simulink model "RotatingMasses_Template"  (R2019b)
settings: Solver=ode1  StartTime=0.0  StopTime=110  FixedStep=0.002  RelTol=1e-3  EnableMultiTasking=on
PostLoadFcn:
  | qc_set_target_type(getConfigSet(bdroot, 'QUARC Default Target Configuration'));
values from neighbouring files (symbols this model uses):
  data = dataset_struct    [create_data.m]    (also in data_loader.m = [])
  deg_to_rad = pi/180    (= 0.0174532925199)    [sensors_parameters.m]
  experiment = merge( experiment, experiment2 )    [blackbox_est.m]    (also in experiment_handler.m = obj.experiments{idx_exp}; guided_script.m = e_h.experiments{40}; test_controllori.m = e_h.load_experiment)
  pulse_to_rad = 2*pi/pulse_per_rev_encoder    (= 0.00153398078789)    [sensors_parameters.m]
  V_th = V_max*1    [sensors_parameters.m]
  Vmin_pot = -4.8924    [sensors_parameters.m]
  volt_to_deg_potentiometer = 352/(Vmax_pot-Vmin_pot)    (= 36.7512711555)    [sensors_parameters.m]
undefined symbols (not defined in the file or in its folder): controller, HIL, qc_get_step_size
libraries: simulink x43, cstblocks x15, quarc_library x5
(part 1 of 3)
settings Model: SimulationMode=external  ExtModeTrigDuration=5000  Creator=CFulford  LastModifiedBy=denniszanutto
settings SolverCC: PositivePriorityOrder=on
settings DataIOCC: LimitDataPoints=on  SaveFormat=Array  SignalLoggingSaveFormat=ModelDataLogs  ReturnWorkspaceOutputs=off
settings OptimizationCC: ExpressionDepthLimit=2147483647  InitFltsAndDblsToZero=on  LifeSpan=inf
settings DebuggingCC: SaveWithParameterizedLinksMsg=none  UnderspecifiedInitializationDetection=Classic  MergeDetectMultiDrivingBlocksExec=none  SolverPrmCheckMsg=warning  MultiTaskDSMMsg=warning  MultiTaskCondExecSysMsg=none  FcnCallInpInsideContextMsg=warning  StateNameClashWarn=warning  SFUnexpectedBacktrackingDiag=warning  SFNoUnconditionalDefaultTransitionDiag=warning  SFExecutionAtInitializationDiag=none  ArithmeticOperatorsInVariantConditions=warning
settings HardwareCC: ProdBitPerPointer=32  ProdBitPerSizeT=32  ProdBitPerPtrDiffT=32  ProdLargestAtomicFloat=None  ProdIntDivRoundTo=Undefined  ProdEndianess=Unspecified  ProdWordSize=32  ProdHWDeviceType=32-bit Generic
settings ModelReferenceCC: PropagateSignalLabelsOutOfModel=off
settings SFSimCC: SimUseLocalCustomCode=off  CustomCodeUndefinedFunction=UseInterfaceOnly
settings RTWCC: Description=QUARC Win64 Target  SystemTargetFile=quarc_win64.tlc  TemplateMakefile=quarc_default_tmf  RTWUseLocalCustomCode=off
settings CodeAppCC: StateflowObjectComments=on
settings STFCustomTargetCC: TargetPreCompLibLocation=C:\PROGRA~3\QUARC\lib\2019b\win64\release  ConcurrentExecutionCompliant=on  GeneratePreprocessorConditionals=Disable all  CombineOutputUpdateFcns=on  CPPClassGenCompliant=on  SystemTargetFile=quarc_win64.tlc
settings GRTTargetCC: TargetPreCompLibLocation=C:\PROGRA~3\QUARC\lib\2019b\win64\release  TargetLangStandard=C89/C90 (ANSI)  ParMdlRefBuildCompliant=off  CompOptLevelCompliant=off  GeneratePreprocessorConditionals=Disable all  MatFileLogging=off  UseToolchainInfoCompliant=off  ExtMode=on  ExtModeMexFile=quarc_comm
settings ConfigComp: CovMetricSettings=dw  CovHtmlReporting=on  CovSaveCumulativeToWorkspaceVar=on  CovSaveSingleToWorkspaceVar=on  CovExternalEMLEnable=off  CovSFcnEnable=off

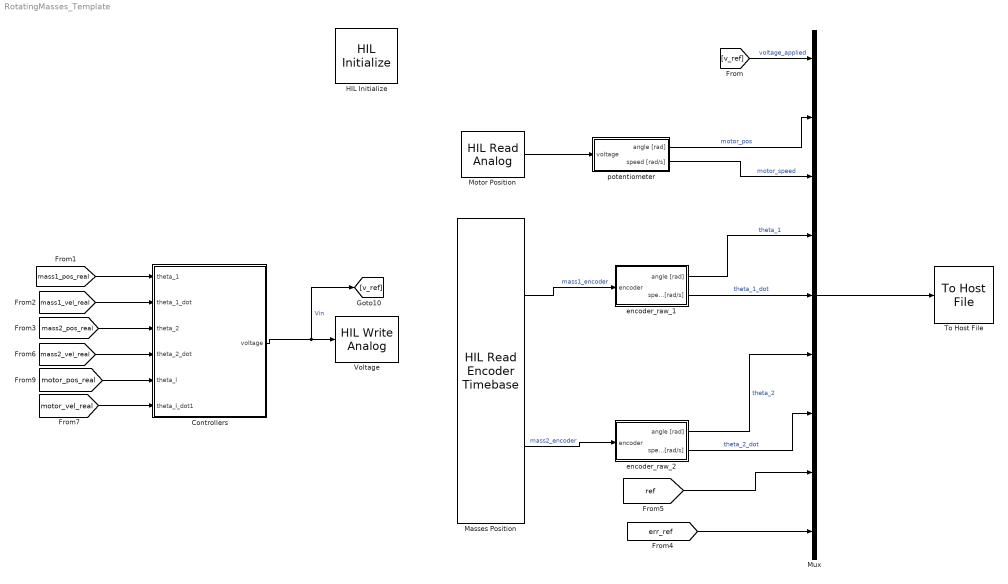
== system RotatingMasses_Template ==
  Controllers : Subsystem
  HIL Initialize : quarc_library/Data Acquisition/Generic/Configuration/HIL Initialize  Priority=-99  object_name=HIL-1  board_type=q2_usb  board_number=0  board_options=d0=digital;d1=digital;led=auto;update_rate=normal;decimation=1  exclusive=off  active=off  hardware_clocks=[0]  clock_modes=[]  initial_clock_frequencies=[]  set_clock_params_at_start=off  set_clock_params_at_switch_in=off  set_clock_frequencies_at_start=off  set_clock_frequencies_at_switch_in=off  analog_input_channels=[0:1]  analog_input_configurations=[]  analog_input_maximums=10  analog_input_minimums=-10  set_analog_input_params_at_start=on  set_analog_input_params_at_switch_in=off  analog_output_channels=[0:1]  analog_output_maximums=10  analog_output_minimums=-10  initial_analog_outputs=[0]  final_analog_outputs=[0]  watchdog_analog_outputs=0  set_analog_output_params_at_start=on  set_analog_output_params_at_switch_in=off  set_analog_outputs_at_start=on  set_analog_outputs_at_switch_in=off  set_analog_outputs_at_terminate=on  set_analog_outputs_at_switch_out=off  set_analog_outputs_on_watchdog=off  digital_input_channels=[]  digital_output_channels=[]  digital_output_configuration=[]  initial_digital_outputs=[1]  final_digital_outputs=[1]  watchdog_digital_outputs=[1]  set_digital_output_params_at_start=off  set_digital_output_params_at_switch_in=off  set_digital_outputs_at_start=on  set_digital_outputs_at_switch_in=off  set_digital_outputs_at_terminate=on  set_digital_outputs_at_switch_out=off  set_digital_outputs_on_watchdog=off  encoder_channels=[0:1]  quadrature=[4]  encoder_filter_frequency=[]  initial_encoder_counts=[0]  set_encoder_params_at_start=on  set_encoder_params_at_switch_in=off  set_encoder_counts_at_start=on  set_encoder_counts_at_switch_in=off  pwm_channels=[]  pwm_modes=[0]  pwm_frequency=1/0.020  pwm_configuration=[]  pwm_alignment=[]  pwm_polarity=[]  pwm_leading_deadband=[]  pwm_trailing_deadband=[]  initial_pwm_outputs=[0]  final_pwm_outputs=[0]  watchdog_pwm_outputs=[0]  set_pwm_params_at_start=on  set_pwm_params_at_switch_in=off  set_pwm_outputs_at_start=on  set_pwm_outputs_at_switch_in=off  set_pwm_outputs_at_terminate=on  set_pwm_outputs_at_switch_out=off  set_pwm_outputs_on_watchdog=off  other_output_channels=[]  initial_other_outputs=[]  final_other_outputs=[]  watchdog_other_outputs=[]  set_other_outputs_at_start=off  set_other_outputs_at_switch_in=off  set_other_outputs_at_terminate=off  set_other_outputs_at_switch_out=off  set_other_outputs_on_watchdog=off
  Masses Position : quarc_library/Data Acquisition/Generic/Timebases/HIL Read Encoder Timebase  object_name=HIL-1  clock=0  channels=[0:1]  samples_in_buffer=max(ceil(1/qc_get_step_size), 1)  active=on  vector_output=off  data_type_mode=Inherit via back propagation  data_type=double
  Motor Position : quarc_library/Data Acquisition/Generic/Immediate I//O/HIL Read Analog  object_name=HIL-1  channels=0  sample_time=qc_get_step_size  active=on  vector_output=off
  Mux : Mux  Inputs=9
  To Host File : quarc_library/Sinks/To Host/To Host File  file_name=data_%{date}_%{time}.mat  variable_name=data_%{date}_%{time}  decimation=1  sample_time=-1  file_format=MAT-file v.5  options=No header or footer  append=off  final_file_name=data_04-May-2021_18-47-16.mat  bitrate=2000000
  Voltage : quarc_library/Data Acquisition/Generic/Immediate I//O/HIL Write Analog  object_name=HIL-1  channels=0  sample_time=-1  active=off  vector_input=off
  encoder_raw_1 : Subsystem
  encoder_raw_2 : Subsystem
  potentiometer : Subsystem
  wires:
  potentiometer/1(angle [rad]) -> Mux/2  "motor_pos"
  Mux/1 -> To Host File/1
  Motor Position/1 -> potentiometer/1(voltage)
  [v_ref] -> Mux/1  "voltage_applied"
  Masses Position/1 -> encoder_raw_1/1(encoder)  "mass1_encoder"
  encoder_raw_1/1("angle [rad] ") -> Mux/4  "theta_1"
  Masses Position/2 -> encoder_raw_2/1(encoder)  "mass2_encoder"
  [err_ref] -> Mux/9
  [ref] -> Mux/8
  ? -> ?
  encoder_raw_1/2(speed [rad/s]) -> Mux/5  "theta_1_dot"
  encoder_raw_2/1("angle [rad] ") -> Mux/6  "theta_2"
  encoder_raw_2/2(speed [rad/s]) -> Mux/7  "theta_2_dot"
  Controllers/1(voltage) -> Voltage/1, [v_ref]  "Vin"
  [mass1_pos_real] -> Controllers/1(theta_1)
  [mass1_vel_real] -> Controllers/2(theta_1_dot)
  [mass2_pos_real] -> Controllers/3(theta_2)
  [mass2_vel_real] -> Controllers/4(theta_2_dot)
  potentiometer/2(speed [rad/s]) -> Mux/3  "motor_speed"
  [motor_pos_real] -> Controllers/5(theta_l)
  [motor_vel_real] -> Controllers/6(theta_l_dot1)

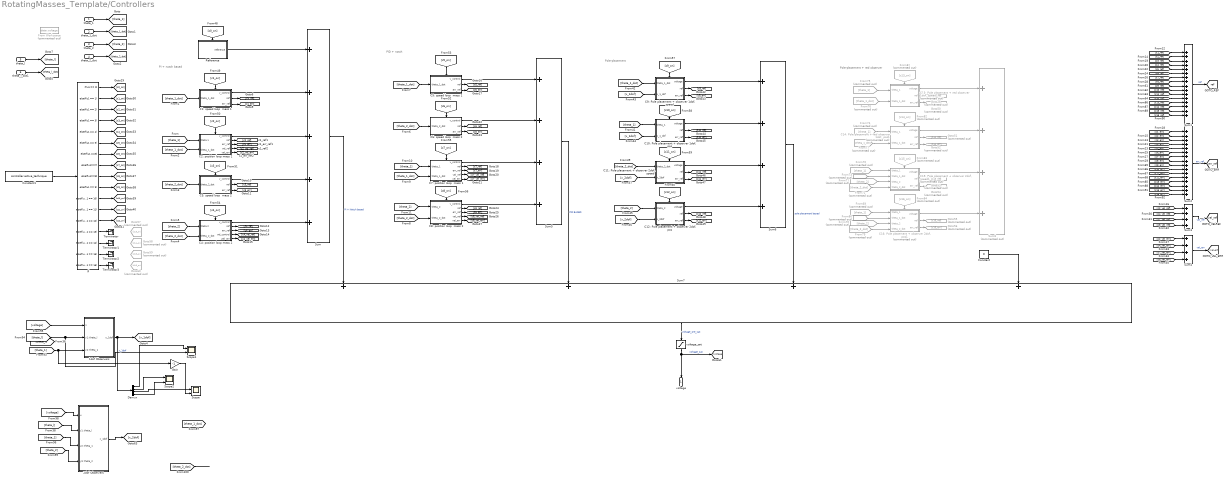
== system RotatingMasses_Template/Controllers ==
  note: Pole-placement
  note: PID + notch
  note: PI + notch based
  note: Pole-placement + red observer
  theta_1 : Inport
  theta_1_dot : Inport  Port=2
  theta_2 : Inport  Port=3
  theta_2_dot : Inport  Port=4
  theta_l : Inport  Port=5
  theta_l_dot1 : Inport  Port=6
  1dof Observers : Subsystem
  2dof Observers : Subsystem
  "C10: Pole placement + observer 1dof, pos" : Subsystem  TreatAsAtomicUnit=on
  "C11: Pole placement + observer 2dof, speed" : Subsystem  TreatAsAtomicUnit=on
  "C12: Pole placement + observer 2dof, pos" : Subsystem  TreatAsAtomicUnit=on
  "C13: Pole placement + red observer 1dof, speed1" : Subsystem  Commented=on  TreatAsAtomicUnit=on
  "C14: Pole placement + red observer 1dof, pos1" : Subsystem  Commented=on  TreatAsAtomicUnit=on
  "C15: Pole placement + observer 2dof, speed1" : Subsystem  Commented=on  TreatAsAtomicUnit=on
  "C16: Pole placement + observer 2dof, pos1" : Subsystem  Commented=on  TreatAsAtomicUnit=on
  C1: speed loop  mass 1 : Subsystem
  C2: position loop mass 1 : Subsystem
  C3: speed loop  mass 2 : Subsystem
  C4: position loop mass 2 : Subsystem
  C5: speed loop  mass 1 : Subsystem
  C6: speed loop  mass 2 : Subsystem
  C7: position loop  mass 1 : Subsystem
  C8: position loop  mass 2 : Subsystem
  "C9: Pole placement + observer 1dof, speed" : Subsystem  TreatAsAtomicUnit=on
  Constant : Constant  Value=0
  Constant1 : Constant  Value=controller.active_technique
  Demux : Demux
  From Workspace : FromWorkspace  Commented=on  VariableName=data.voltage  SampleTime=0
  From{69..70,74..75} (4 alike) : From  Commented=on  GotoTag=theta_1
  From71 : From  Commented=on  GotoTag=theta_2
  From72 : From  Commented=on  GotoTag=theta_2_dot
  From{73,76..77,80} (4 alike) : From  Commented=on  GotoTag=theta_1_dot
  From78 : From  Commented=on  GotoTag=theta_2
  From79 : From  Commented=on  GotoTag=theta_2_dot
  From81 : From  Commented=on  GotoTag=c13_on
  From82 : From  Commented=on  GotoTag=c14_on
  From83 : From  Commented=on  GotoTag=c15_on
  From84 : From  Commented=on  GotoTag=c16_on
  Gain : Gain  Gain=-1
  Goto28 : Goto  Commented=on  GotoTag=c13_ref
  Goto50 : Goto  Commented=on  GotoTag=c13_err
  Goto51 : Goto  Commented=on  GotoTag=c14_ref
  Goto52 : Goto  Commented=on  GotoTag=c14_err
  Goto53 : Goto  Commented=on  GotoTag=c15_ref
  Goto54 : Goto  Commented=on  GotoTag=c15_err
  Goto55 : Goto  Commented=on  GotoTag=c16_ref
  Goto56 : Goto  Commented=on  GotoTag=c16_err
  Goto57 : Goto  Commented=on  GotoTag=c13_on
  Goto58 : Goto  Commented=on  GotoTag=c14_on
  Goto59 : Goto  Commented=on  GotoTag=c15_on
  Goto60 : Goto  Commented=on  GotoTag=c16_on
  If : If  IfExpression=u1 == 0  ElseIfExpressions=u1 == 1, u1 == 2, u1 == 3, u1 == 4, u1 == 5, u1 ==6, u1==7, u1==8, u1 == 9, u1 == 10, u1 == 11, u1 == 12, u1 == 13, u1 == 14, u1 == 15, u1 == 16  ShowElse=off
  Reference : Subsystem
  Scope : Scope  NumInputPorts=2
  Scope1 : Scope  NumInputPorts=2
  Scope2 : Scope  NumInputPorts=2
  Sum : Sum  Inputs=+++++
  Sum1 : Sum  Inputs=++++++++++++++++
  Sum2 : Sum  Inputs=++++++++++++++++
  Sum{3..7} (5 alike) : Sum  Inputs=++++
  Sum8 : Sum  Commented=on  Inputs=++++
  Terminator{,1..3} (4 alike) : Terminator
  voltage_sat : Saturate  UpperLimit=V_th  LowerLimit=-V_th
  voltage : Outport
  tag scope: err_ref=global, ref=global, vel_ref=global
  wires:
  voltage_sat/1 -> voltage/1, [voltage]  "voltage_sat"
  theta_1_dot/1 -> [theta_1_dot]
  C4: position loop mass 2/1(v_control) -> Sum/5
  C3: speed loop  mass 2/1(v_control) -> Sum/4
  C2: position loop mass 1/1(v_control) -> Sum/3
  C1: speed loop  mass 1/1(v_control) -> Sum/2
  Reference/1(reference) -> Sum/1
  If/1 -> [c0_on]
  Constant1/1 -> If/1
  theta_1/1 -> [theta_1]
  [theta_1_dot] -> C1: speed loop  mass 1/1(theta_1_dot)
  [theta_1_dot] -> C2: position loop mass 1/2(theta_1_dot)
  [theta_1] -> C2: position loop mass 1/1(theta 1)
  theta_2_dot/1 -> [theta_2_dot]
  [theta_2_dot] -> C3: speed loop  mass 2/1(theta_2_dot)
  [theta_2_dot] -> C4: position loop mass 2/2(theta_2_dot)
  theta_2/1 -> [theta_2]
  [theta_2] -> C4: position loop mass 2/1(theta 2)
  [theta_2_dot] -> C6: speed loop  mass 2/1(theta_2_dot)
  C6: speed loop  mass 2/1(v_control) -> Sum5/2
  C5: speed loop  mass 1/1(v_control) -> Sum5/1
  [theta_1_dot] -> C5: speed loop  mass 1/1(theta_1_dot)
  C8: position loop  mass 2/1(v_control) -> Sum5/4
  [theta_1_dot] -> C7: position loop  mass 1/2(theta_1_dot)
  [theta_2_dot] -> C8: position loop  mass 2/2(theta_2_dot)
  C7: position loop  mass 1/1(v_control) -> Sum5/3
  [theta_1] -> C7: position loop  mass 1/1(theta_1)
  [theta_2] -> C8: position loop  mass 2/1(theta_2)
  C1: speed loop  mass 1/2("ref ") -> [c1_ref]
  C1: speed loop  mass 1/3("err_ref ") -> [c1_err]
  C2: position loop mass 1/5("vel_err ") -> [c2_vel_err]
  C2: position loop mass 1/4("vel_ref ") -> [c2_vel_ref]
  C2: position loop mass 1/3("err_ref ") -> [c2_err]
  C3: speed loop  mass 2/2("ref ") -> [c3_ref]
  C3: speed loop  mass 2/3("err_ref ") -> [c3_err]
  C4: position loop mass 2/3(err_ref) -> [c4_err]
  C4: position loop mass 2/2(ref) -> [c4_ref]
  C4: position loop mass 2/4(vel_control) -> [c4_vel_ref]
  C4: position loop mass 2/5("vell_err ") -> [c4_vel_err]
  C5: speed loop  mass 1/2("ref ") -> [c5_ref]
  C5: speed loop  mass 1/3("err_ref ") -> [c5_err]
  C7: position loop  mass 1/5(vel_err) -> [c7_vel_err]
  C7: position loop  mass 1/2("ref ") -> [c7_ref]
  C7: position loop  mass 1/3("err_ref ") -> [c7_err]
  C7: position loop  mass 1/4(vel_ref) -> [c7_vel_ref]
  C6: speed loop  mass 2/2("ref ") -> [c6_ref]
  C6: speed loop  mass 2/3("err_ref ") -> [c6_err]
  C8: position loop  mass 2/2("ref ") -> [c8_ref]
  C8: position loop  mass 2/3("err_ref ") -> [c8_err]
  C8: position loop  mass 2/4(vel_ref) -> [c8_vel_ref]
  C8: position loop  mass 2/5(vel_err) -> [c8_vel_err]
  [c1_ref] -> Sum1/1
  [c2_ref] -> Sum1/2
  Sum1/1 -> [ref]  "ref"
  [c1_err] -> Sum2/1
  Sum2/1 -> [err_ref]  "err_ref"
  [c2_err] -> Sum2/2
  C2: position loop mass 1/2("ref ") -> [c2_ref]
  [c3_err] -> Sum2/3
  [c3_ref] -> Sum1/3
  [c6_err] -> Sum2/6
  [c7_err] -> Sum2/7
  [c8_err] -> Sum2/8
  [c4_err] -> Sum2/4
  [c5_err] -> Sum2/5
  [c4_ref] -> Sum1/4
  [c5_ref] -> Sum1/5
  [c6_ref] -> Sum1/6
  [c8_ref] -> Sum1/8
  [c7_ref] -> Sum1/7
  [c8_vel_ref] -> Sum3/4
  [c7_vel_ref] -> Sum3/3
  [c4_vel_ref] -> Sum3/2
  [c2_vel_ref] -> Sum3/1
  Sum3/1 -> [vel_ref]  "vel_ref"
  [c2_vel_err] -> Sum4/1
  Sum4/1 -> [vel_err]  "vel_err"
  [c4_vel_err] -> Sum4/2
  [c7_vel_err] -> Sum4/3
  [c8_vel_err] -> Sum4/4
  [theta_2_dot] -> "C11: Pole placement + observer 2dof, speed"/1(theta_2_dot)
  "C9: Pole placement + observer 1dof, speed"/1(voltage) -> Sum6/1
  [theta_1_dot] -> "C9: Pole placement + observer 1dof, speed"/1(theta_1_dot)
  [x_1dof] -> "C9: Pole placement + observer 1dof, speed"/2(x_1_dof)
  [theta_1] -> "C10: Pole placement + observer 1dof, pos"/1(theta_1)
  [x_1dof] -> "C10: Pole placement + observer 1dof, pos"/2(x_1_dof)
  "C10: Pole placement + observer 1dof, pos"/1(voltage) -> Sum6/2
  "C11: Pole placement + observer 2dof, speed"/1(voltage) -> Sum6/3
  "C12: Pole placement + observer 2dof, pos"/1(voltage) -> Sum6/4
  [x_2dof] -> "C12: Pole placement + observer 2dof, pos"/2(x_2dof)
  [theta_2] -> "C12: Pole placement + observer 2dof, pos"/1(theta_2)
  [c0_on] -> Reference/Action
  If/2 -> [c1_on]
  [c1_on] -> C1: speed loop  mass 1/Action
  If/3 -> [c2_on]
  [c2_on] -> C2: position loop mass 1/Action
  If/4 -> [c3_on]
  [c3_on] -> C3: speed loop  mass 2/Action
  If/7 -> [c6_on]
  If/6 -> [c5_on]
  If/5 -> [c4_on]
  [c4_on] -> C4: position loop mass 2/Action
  [c5_on] -> C5: speed loop  mass 1/Action
  [c6_on] -> C6: speed loop  mass 2/Action
  If/8 -> [c7_on]
  [c7_on] -> C7: position loop  mass 1/Action
  If/9 -> [c8_on]
  [c8_on] -> C8: position loop  mass 2/Action
  If/10 -> [c9_on]
  [c9_on] -> "C9: Pole placement + observer 1dof, speed"/Action
  If/11 -> [c10_on]
  [c10_on] -> "C10: Pole placement + observer 1dof, pos"/Action
  If/12 -> [c11_on]
  [c11_on] -> "C11: Pole placement + observer 2dof, speed"/Action
  [c12_on] -> "C12: Pole placement + observer 2dof, pos"/Action
  If/13 -> [c12_on]
  "C9: Pole placement + observer 1dof, speed"/2(ref) -> [c9_ref]
  "C9: Pole placement + observer 1dof, speed"/3(err_ref) -> [c9_err]
  "C10: Pole placement + observer 1dof, pos"/2(ref) -> [c10_ref]
  "C10: Pole placement + observer 1dof, pos"/3(err_ref) -> [c10_err]
  "C11: Pole placement + observer 2dof, speed"/2(ref) -> [c11_ref]
  "C11: Pole placement + observer 2dof, speed"/3(err_ref) -> [c11_err]
  "C12: Pole placement + observer 2dof, pos"/2(ref) -> [c12_ref]
  "C12: Pole placement + observer 2dof, pos"/3(err_ref) -> [c12_err]
  [c9_ref] -> Sum1/9
  [c10_ref] -> Sum1/10
  [c11_ref] -> Sum1/11
  [c12_ref] -> Sum1/12
  [c9_err] -> Sum2/9
  [c10_err] -> Sum2/10
  [c11_err] -> Sum2/11
  [c12_err] -> Sum2/12
  "C15: Pole placement + observer 2dof, speed1"/3(err_ref) -> Goto54/1
  "C16: Pole placement + observer 2dof, pos1"/2(ref) -> Goto55/1
  From84/1 -> "C16: Pole placement + observer 2dof, pos1"/Action
  From71/1 -> "C15: Pole placement + observer 2dof, speed1"/3(theta_2)
  "C16: Pole placement + observer 2dof, pos1"/3(err_ref) -> Goto56/1
  "C13: Pole placement + red observer 1dof, speed1"/2(ref) -> Goto28/1
  From78/1 -> "C16: Pole placement + observer 2dof, pos1"/3(theta_2)
  From74/1 -> "C14: Pole placement + red observer 1dof, pos1"/1(theta_1)
  "C13: Pole placement + red observer 1dof, speed1"/3(err_ref) -> Goto50/1
  "C14: Pole placement + red observer 1dof, pos1"/3(err_ref) -> Goto52/1
  From79/1 -> "C16: Pole placement + observer 2dof, pos1"/4(theta_2_dot)
  From80/1 -> "C16: Pole placement + observer 2dof, pos1"/2(theta_1_dot)
  From75/1 -> "C13: Pole placement + red observer 1dof, speed1"/1(theta_1)
  From69/1 -> "C16: Pole placement + observer 2dof, pos1"/1(theta_1)
  From76/1 -> "C13: Pole placement + red observer 1dof, speed1"/2(theta_1_dot)
  "C15: Pole placement + observer 2dof, speed1"/2(ref) -> Goto53/1
  From83/1 -> "C15: Pole placement + observer 2dof, speed1"/Action
  From70/1 -> "C15: Pole placement + observer 2dof, speed1"/1(theta_1)
  "C13: Pole placement + red observer 1dof, speed1"/1(voltage) -> Sum8/1
  "C14: Pole placement + red observer 1dof, pos1"/2(ref) -> Goto51/1
  From77/1 -> "C14: Pole placement + red observer 1dof, pos1"/2(theta_1_dot)
  From73/1 -> "C15: Pole placement + observer 2dof, speed1"/2(theta_1_dot)
  From72/1 -> "C15: Pole placement + observer 2dof, speed1"/4(theta_2_dot)
  "C15: Pole placement + observer 2dof, speed1"/1(voltage) -> Sum8/3
  "C16: Pole placement + observer 2dof, pos1"/1(voltage) -> Sum8/4
  "C14: Pole placement + red observer 1dof, pos1"/1(voltage) -> Sum8/2
  From81/1 -> "C13: Pole placement + red observer 1dof, speed1"/Action
  From82/1 -> "C14: Pole placement + red observer 1dof, pos1"/Action
  [c13_err] -> Sum2/13
  [c13_ref] -> Sum1/13
  [c14_ref] -> Sum1/14
  [c14_err] -> Sum2/14
  [c15_ref] -> Sum1/15
  [c16_ref] -> Sum1/16
  [c15_err] -> Sum2/15
  [c16_err] -> Sum2/16
  Sum/1 -> Sum7/1  "PI + Notch based"
  Sum5/1 -> Sum7/2  "PID BASED"
  Sum6/1 -> Sum7/3  "pole placement based"
  [voltage] -> 2dof Observers/1("u ")
  [theta_l] -> 2dof Observers/2(y1: theta_l)
  [theta_1] -> 2dof Observers/3(y2: theta_1)
  [theta_2] -> 2dof Observers/4(y3: theta_2)
  [theta_2_dot] -> ?
  [x_2dof] -> "C11: Pole placement + observer 2dof, speed"/2(x_2dof)
  Constant/1 -> Sum7/4
  If/14 -> Terminator/1
  If/15 -> Terminator1/1
  If/16 -> Terminator2/1
  If/17 -> Terminator3/1
  [theta_l] -> Scope1/2, 1dof Observers/2(y1: theta_l)
  [theta_1] -> Gain/1, 1dof Observers/3(y2: theta_1)
  Demux/2 -> Scope2/1
  Sum7/1 -> voltage_sat/1  "voltage_pre_sat"
  [voltage] -> 1dof Observers/1(u)
  1dof Observers/1(x_1dof) -> Demux/1, [x_1dof]  "x_1dof"
  Demux/1 -> Scope1/1
  Demux/4 -> Scope2/2
  Demux/3 -> Scope/1
  Gain/1 -> Scope/2
  theta_l_dot1/1 -> [theta_l_dot]
  theta_l/1 -> [theta_l]
  2dof Observers/1(x_1dof) -> [x_2dof]

== system RotatingMasses_Template/encoder_raw_1 ==
  encoder : Inport
  Discrete Derivative1 : simulink/Discrete/Discrete Derivative  gainval=1  ICPrevScaledInput=0.0  OutMin=[]  OutMax=[]  OutDataType=fixdt(1, 16)  OutScaling=2^-10  DoSatur=off
  Gain3 : Gain  Gain=pulse_to_rad
  "Reset and buffer count " : MATLAB Function  TreatAsAtomicUnit=on
  Sum : Sum  Inputs=++|
  Transfer Fcn1 : TransferFcn  Numerator=[experiment.w_filter]  Denominator=[1 experiment.w_filter]
  "angle [rad] " : Outport
  speed [rad/s] : Outport  Port=2
  tag scope: mass1_pos_real=global, mass1_vel_real=global
  wires:
  encoder/1 -> "Reset and buffer count "/1(u)  "buffer_value"
  "Reset and buffer count "/1(y) -> Gain3/1
  Gain3/1 -> Sum/2, Discrete Derivative1/1  "relative_mov_rad"
  Discrete Derivative1/1 -> Transfer Fcn1/1  "istantaneous_speed"
  Transfer Fcn1/1 -> [mass1_vel_real], speed [rad/s]/1  "filtered_speed"
  Sum/1 -> [mass1_pos_real], "angle [rad] "/1
  [starting_position] -> Sum/1

== system RotatingMasses_Template/encoder_raw_2 ==
  encoder : Inport
  Discrete Derivative1 : simulink/Discrete/Discrete Derivative  gainval=1  ICPrevScaledInput=0.0  OutMin=[]  OutMax=[]  OutDataType=fixdt(1, 16)  OutScaling=2^-10  DoSatur=off
  Gain3 : Gain  Gain=pulse_to_rad
  "Reset and buffer count " : MATLAB Function  TreatAsAtomicUnit=on
  Sum : Sum  Inputs=++|
  Transfer Fcn1 : TransferFcn  Numerator=[experiment.w_filter]  Denominator=[1 experiment.w_filter]
  "angle [rad] " : Outport
  speed [rad/s] : Outport  Port=2
  tag scope: mass2_pos_real=global, mass2_vel_real=global
  wires:
  encoder/1 -> "Reset and buffer count "/1(u)  "buffer_value"
  "Reset and buffer count "/1(y) -> Gain3/1
  Gain3/1 -> Sum/2, Discrete Derivative1/1  "relative_mov_rad"
  Discrete Derivative1/1 -> Transfer Fcn1/1  "istantaneous_speed"
  Transfer Fcn1/1 -> [mass2_vel_real], speed [rad/s]/1  "filtered_speed"
  Sum/1 -> [mass2_pos_real], "angle [rad] "/1
  [starting_position] -> Sum/1

== system RotatingMasses_Template/potentiometer ==
  voltage : Inport
  Constant : Constant  Value=-Vmin_pot
  Constant1 : Constant  Value=352/2
  Discrete Derivative : simulink/Discrete/Discrete Derivative  gainval=1  ICPrevScaledInput=0.0  OutMin=[]  OutMax=[]  OutDataType=fixdt(1, 16)  OutScaling=2^-10  DoSatur=off
  Starting position : MATLAB Function  TreatAsAtomicUnit=on  SystemSampleTime=0.002
  Sum : Sum  Inputs=|++
  Sum1 : Sum  Inputs=++|
  conversion_deg_rad : Gain  Gain=deg_to_rad
  conversion_v_deg : Gain  Gain=volt_to_deg_potentiometer
  angle [rad] : Outport
  speed [rad/s] : Outport  Port=2
  tag scope: motor_pos_real=global, motor_vel_real=global, starting_position=global
  wires:
  Constant/1 -> Sum/2  "v_min"
  voltage/1 -> Sum/1  "v_in"
  Sum1/1 -> conversion_deg_rad/1  "deg"
  Sum/1 -> conversion_v_deg/1  "v_0_10"
  Discrete Derivative/1 -> [motor_vel_real], speed [rad/s]/1  "motor_vel"
  conversion_deg_rad/1 -> Starting position/1(u), Discrete Derivative/1, [motor_pos_real], angle [rad]/1
  conversion_v_deg/1 -> Sum1/2  "deg"
  Constant1/1 -> Sum1/1
  Starting position/1(y) -> [starting_position]

== system RotatingMasses_Template/Controllers/1dof Observers ==
  u : Inport
  y1: theta_l : Inport  Port=2
  y2: theta_1 : Inport  Port=3
  Constant : Constant  Value=controller.active_observer
  Constant2 : Constant  Value=0
  MATLAB Function1 : MATLAB Function  TreatAsAtomicUnit=on  SystemSampleTime=0.002
  Mux : Mux
  Red_obs_1dof : Subsystem  Commented=on
  Sum : Sum  Inputs=++|
  Sum9 : Sum  Inputs=-+|
  Switch : Switch  Threshold=1
  obs_1_dof : Subsystem
  x_1dof : Outport
  wires:
  Sum9/1 -> Red_obs_1dof/2(y1: theta_l), obs_1_dof/2(y1: theta_l)
  y2: theta_1/1 -> Red_obs_1dof/3(y2: theta_1), obs_1_dof/3(y2: theta_1)
  Constant/1 -> Switch/2
  u/1 -> Red_obs_1dof/1(u), obs_1_dof/1(u)
  Sum/1 -> x_1dof/1
  Red_obs_1dof/1(x) -> Switch/1
  obs_1_dof/1(x) -> Switch/3
  MATLAB Function1/1(y) -> Mux/3, Mux/1, Sum9/1
  Mux/1 -> Sum/1
  Constant2/1 -> Mux/4, Mux/2
  Switch/1 -> Sum/2
  y1: theta_l/1 -> MATLAB Function1/1(u), Sum9/2

== system RotatingMasses_Template/Controllers/2dof Observers ==
  "u " : Inport
  y1: theta_l : Inport  Port=2
  y2: theta_1 : Inport  Port=3
  y3: theta_2 : Inport  Port=4
  Constant1 : Constant  Value=controller.active_observer
  Constant2 : Constant  Value=0
  MATLAB Function1 : MATLAB Function  TreatAsAtomicUnit=on  SystemSampleTime=0.002
  Mux : Mux  Inputs=6
  Observer_2dof : Subsystem
  Sum : Sum  Inputs=++|
  Sum1 : Sum  Inputs=-+|
  Switch1 : Switch  Threshold=1
  red_obs_2dof : Subsystem  Commented=on
  x_1dof : Outport
  wires:
  y3: theta_2/1 -> red_obs_2dof/4(y3: theta_2), Observer_2dof/4(y3: theta_2)
  y2: theta_1/1 -> red_obs_2dof/3(y2: theta_1_dot), Observer_2dof/3(y2: theta_1)
  "u "/1 -> Observer_2dof/1(u), red_obs_2dof/1(u)
  Sum/1 -> x_1dof/1
  Switch1/1 -> Sum/2
  MATLAB Function1/1(y) -> Mux/5, Mux/3, Mux/1, Sum1/1
  Constant2/1 -> Mux/6, Mux/4, Mux/2
  Mux/1 -> Sum/1
  Observer_2dof/1(x_2_dof) -> Switch1/3
  red_obs_2dof/1(x_2dof) -> Switch1/1
  Constant1/1 -> Switch1/2
  Sum1/1 -> Observer_2dof/2(y1: theta_l), red_obs_2dof/2(y1: theta_1)
  y1: theta_l/1 -> Sum1/2, MATLAB Function1/1(u)

== system RotatingMasses_Template/Controllers/C10: Pole placement + observer 1dof, pos ==
  theta_1 : Inport
  x_1_dof : Inport  Port=2
  Action Port : ActionPort  ActionPortLabel=elseif( u1 == 10)
  K_v : Gain  Gain=controller.c10.K_v
  Pole placement : Gain  Gain=controller.c10.K_x  Multiplication=Matrix(K*u)
  Reference : Subsystem
  Sum : Sum  Inputs=--|
  Sum2 : Sum  Inputs=|+-
  voltage : Outport
  ref : Outport  Port=2
  err_ref : Outport  Port=3
  wires:
  Pole placement/1 -> Sum/2  "voltage_pp"
  Sum/1 -> voltage/1
  K_v/1 -> Sum/1  "voltage_closed-loop"
  Sum2/1 -> err_ref/1, K_v/1  "err_ref"
  Reference/1(reference) -> ref/1, Sum2/1
  theta_1/1 -> Sum2/2
  x_1_dof/1 -> Pole placement/1

== system RotatingMasses_Template/Controllers/C11: Pole placement + observer 2dof, speed ==
  theta_2_dot : Inport
  x_2dof : Inport  Port=2
  Action Port : ActionPort  ActionPortLabel=elseif( u1 == 11)
  Integrator : Integrator
  K_v : Gain  Gain=controller.c11.K_v
  Pole placement : Gain  Gain=controller.c11.K_x  Multiplication=Matrix(K*u)
  Reference : Subsystem
  Sum : Sum  Inputs=--|
  Sum2 : Sum  Inputs=|+-
  voltage : Outport
  ref : Outport  Port=2
  err_ref : Outport  Port=3
  wires:
  Pole placement/1 -> Sum/2  "voltage_pp"
  Sum/1 -> voltage/1
  K_v/1 -> Sum/1  "voltage_closed-loop"
  Integrator/1 -> K_v/1
  Sum2/1 -> Integrator/1, err_ref/1  "err_ref"
  Reference/1(reference) -> Sum2/1, ref/1
  theta_2_dot/1 -> Sum2/2
  x_2dof/1 -> Pole placement/1

== system RotatingMasses_Template/Controllers/C12: Pole placement + observer 2dof, pos ==
  theta_2 : Inport
  x_2dof : Inport  Port=2
  Action Port : ActionPort  ActionPortLabel=elseif( u1 == 12)
  K_v : Gain  Gain=controller.c12.K_v
  Pole placement : Gain  Gain=controller.c12.K_x  Multiplication=Matrix(K*u)
  Reference : Subsystem
  Sum : Sum  Inputs=--|
  Sum2 : Sum  Inputs=|+-
  voltage : Outport
  ref : Outport  Port=2
  err_ref : Outport  Port=3
  wires:
  Pole placement/1 -> Sum/2  "voltage_pp"
  Sum/1 -> voltage/1
  K_v/1 -> Sum/1  "voltage_closed-loop"
  Sum2/1 -> err_ref/1, K_v/1  "err_ref"
  Reference/1(reference) -> ref/1, Sum2/1
  theta_2/1 -> Sum2/2
  x_2dof/1 -> Pole placement/1

== system RotatingMasses_Template/Controllers/C13: Pole placement + red observer 1dof, speed1 ==
  theta_1 : Inport
  theta_1_dot : Inport  Port=2
  Action Port : ActionPort
  Integrator : Integrator
  K_v : Gain  Gain=controller.c13.K_v
  K_x : Gain  Gain=controller.c13.K_x  Multiplication=Matrix(K*u)
  Red_obs_1dof : Subsystem
  Reference : Subsystem
  Saturation : Saturate  UpperLimit=V_th  LowerLimit=-V_th
  Sum : Sum  Inputs=--|
  Sum2 : Sum  Inputs=|+-
  voltage : Outport
  ref : Outport  Port=2
  err_ref : Outport  Port=3
  wires:
  Saturation/1 -> Red_obs_1dof/2(In2), voltage/1
  Sum/1 -> Saturation/1
  K_v/1 -> Sum/1  "voltage_closed-loop"
  Integrator/1 -> K_v/1
  Sum2/1 -> err_ref/1, Integrator/1  "err_ref"
  Reference/1(reference) -> ref/1, Sum2/1
  K_x/1 -> Sum/2
  theta_1_dot/1 -> Red_obs_1dof/3(In3), Sum2/2
  theta_1/1 -> Red_obs_1dof/1(In1)
  Red_obs_1dof/1(x) -> K_x/1

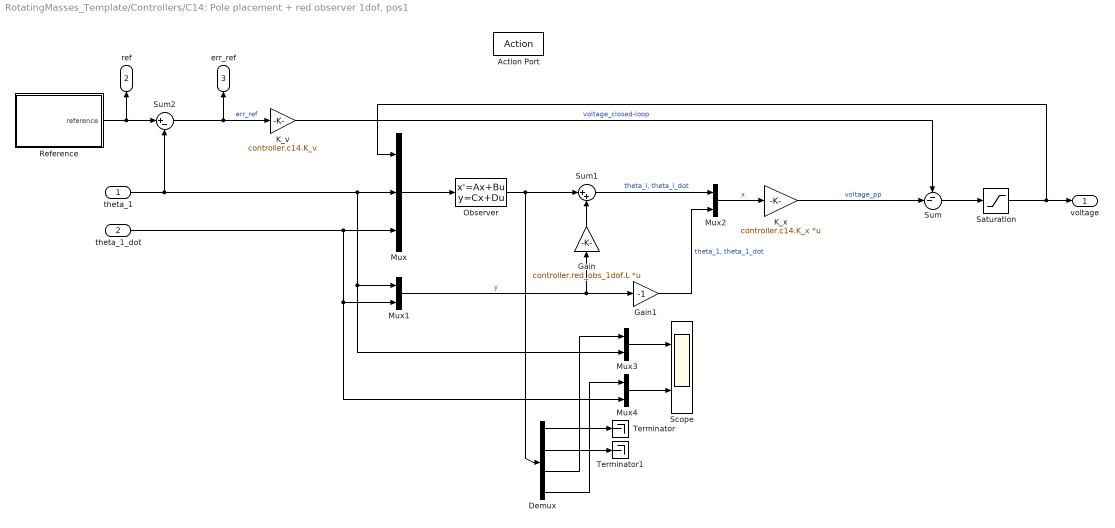
== system RotatingMasses_Template/Controllers/C14: Pole placement + red observer 1dof, pos1 ==
  theta_1 : Inport
  theta_1_dot : Inport  Port=2
  Action Port : ActionPort
  Demux : Demux
  Gain : Gain  Gain=controller.red_obs_1dof.L  Multiplication=Matrix(K*u)
  Gain1 : Gain  Gain=-1
  K_v : Gain  Gain=controller.c14.K_v
  K_x : Gain  Gain=controller.c14.K_x  Multiplication=Matrix(K*u)
  Mux : Mux  Inputs=3
  Mux{1..4} (4 alike) : Mux  Inputs=2
  Observer : StateSpace  A=controller.red_obs_1dof.A  B=controller.red_obs_1dof.B  C=controller.red_obs_1dof.C  D=controller.red_obs_1dof.D  InitialCondition=[data.motor_pos_0;0]
  Reference : Subsystem
  Saturation : Saturate  UpperLimit=V_th  LowerLimit=-V_th
  Scope : Scope  NumInputPorts=2
  Sum : Sum  Inputs=--|
  Sum1 : Sum  Inputs=|++
  Sum2 : Sum  Inputs=|+-
  Terminator : Terminator
  Terminator1 : Terminator
  voltage : Outport
  ref : Outport  Port=2
  err_ref : Outport  Port=3
  wires:
  Saturation/1 -> Mux/1, voltage/1
  Sum/1 -> Saturation/1
  K_v/1 -> Sum/1  "voltage_closed-loop"
  Sum2/1 -> err_ref/1, K_v/1  "err_ref"
  Reference/1(reference) -> ref/1, Sum2/1
  Mux2/1 -> K_x/1  "x"
  Mux/1 -> Observer/1
  Gain/1 -> Sum1/2
  Sum1/1 -> Mux2/1  "theta_l, theta_l_dot"
  Gain1/1 -> Mux2/2  "theta_1, theta_1_dot"
  Mux1/1 -> Gain/1, Gain1/1  "y"
  K_x/1 -> Sum/2  "voltage_pp"
  theta_1/1 -> Mux/2, Mux3/2, Mux1/1, Sum2/2
  Demux/2 -> Terminator1/1
  theta_1_dot/1 -> Mux/3, Mux4/2, Mux1/2
  Demux/1 -> Terminator/1
  Mux3/1 -> Scope/1
  Observer/1 -> Sum1/1, Demux/1
  Demux/4 -> Mux4/1
  Demux/3 -> Mux3/1
  Mux4/1 -> Scope/2

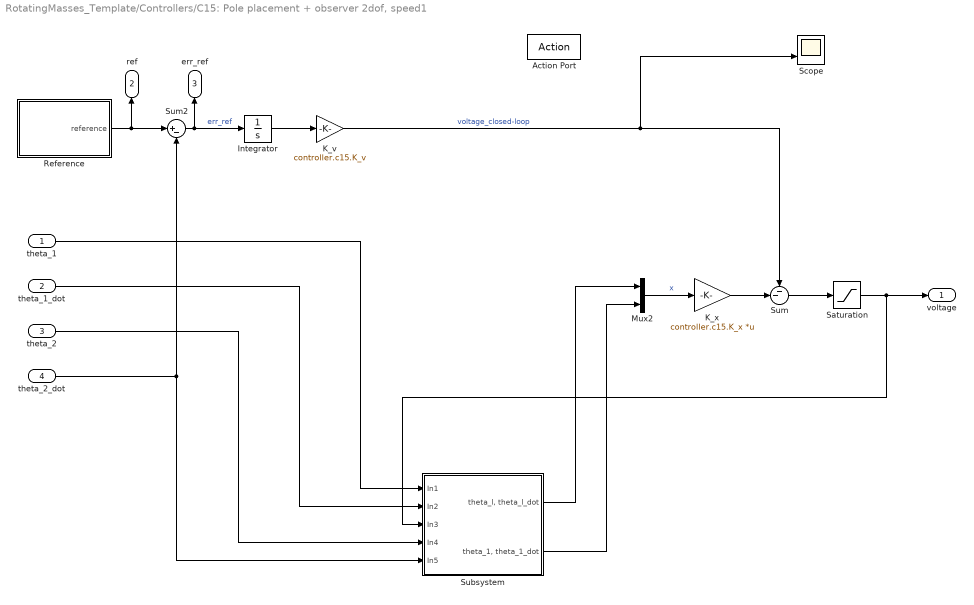
== system RotatingMasses_Template/Controllers/C15: Pole placement + observer 2dof, speed1 ==
  theta_1 : Inport
  theta_1_dot : Inport  Port=2
  theta_2 : Inport  Port=3
  theta_2_dot : Inport  Port=4
  Action Port : ActionPort
  Integrator : Integrator
  K_v : Gain  Gain=controller.c15.K_v
  K_x : Gain  Gain=controller.c15.K_x  Multiplication=Matrix(K*u)
  Mux2 : Mux  Inputs=2
  Reference : Subsystem
  Saturation : Saturate  UpperLimit=V_th  LowerLimit=-V_th
  Scope : Scope  NumInputPorts=2
  Subsystem : Subsystem
  Sum : Sum  Inputs=--|
  Sum2 : Sum  Inputs=|+-
  voltage : Outport
  ref : Outport  Port=2
  err_ref : Outport  Port=3
  wires:
  Sum/1 -> Saturation/1
  K_v/1 -> Scope/2, Sum/1  "voltage_closed-loop"
  Integrator/1 -> K_v/1
  Sum2/1 -> Integrator/1, err_ref/1  "err_ref"
  Reference/1(reference) -> Sum2/1, ref/1
  Mux2/1 -> K_x/1  "x"
  Saturation/1 -> Subsystem/3(In3), voltage/1
  K_x/1 -> Sum/2
  theta_2_dot/1 -> Subsystem/5(In5), Sum2/2
  theta_1/1 -> Subsystem/1(In1)
  theta_1_dot/1 -> Subsystem/2(In2)
  theta_2/1 -> Subsystem/4(In4)
  Subsystem/1("theta_l, theta_l_dot") -> Mux2/1
  Subsystem/2("theta_1, theta_1_dot") -> Mux2/2

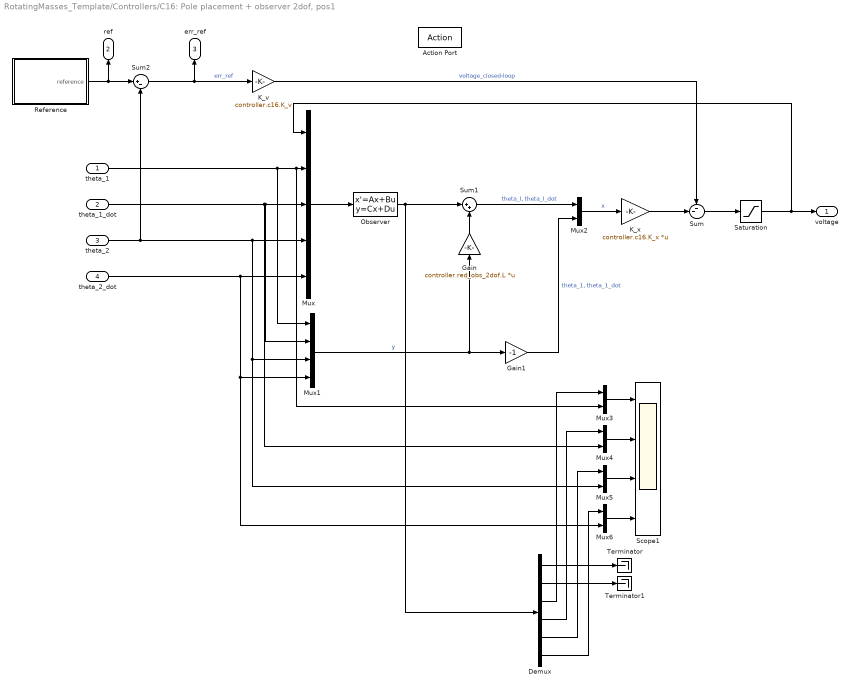
== system RotatingMasses_Template/Controllers/C16: Pole placement + observer 2dof, pos1 ==
  theta_1 : Inport
  theta_1_dot : Inport  Port=2
  theta_2 : Inport  Port=3
  theta_2_dot : Inport  Port=4
  Action Port : ActionPort
  Demux : Demux  Outputs=6
  Gain : Gain  Gain=controller.red_obs_2dof.L  Multiplication=Matrix(K*u)
  Gain1 : Gain  Gain=-1
  K_v : Gain  Gain=controller.c16.K_v
  K_x : Gain  Gain=controller.c16.K_x  Multiplication=Matrix(K*u)
  Mux : Mux  Inputs=5
  Mux1 : Mux
  Mux{2..6} (5 alike) : Mux  Inputs=2
  Observer : StateSpace  A=controller.red_obs_2dof.A  B=controller.red_obs_2dof.B  C=controller.red_obs_2dof.C  D=controller.red_obs_2dof.D  InitialCondition=[data.motor_pos_0;0]
  Reference : Subsystem
  Saturation : Saturate  UpperLimit=V_th  LowerLimit=-V_th
  Scope1 : Scope  NumInputPorts=4
  Sum : Sum  Inputs=--|
  Sum1 : Sum  Inputs=|++
  Sum2 : Sum  Inputs=|+-
  Terminator : Terminator
  Terminator1 : Terminator
  voltage : Outport
  ref : Outport  Port=2
  err_ref : Outport  Port=3
  wires:
  Sum2/1 -> err_ref/1, K_v/1  "err_ref"
  Reference/1(reference) -> ref/1, Sum2/1
  Sum1/1 -> Mux2/1  "theta_l, theta_l_dot"
  Mux1/1 -> Gain/1, Gain1/1  "y"
  Gain/1 -> Sum1/2
  Mux/1 -> Observer/1
  Gain1/1 -> Mux2/2  "theta_1, theta_1_dot"
  Mux2/1 -> K_x/1  "x"
  Saturation/1 -> Mux/1, voltage/1
  K_v/1 -> Sum/1  "voltage_closed-loop"
  K_x/1 -> Sum/2
  Sum/1 -> Saturation/1
  Demux/3 -> Mux3/1
  Demux/1 -> Terminator/1
  Mux4/1 -> Scope1/2
  Mux5/1 -> Scope1/3
  theta_1_dot/1 -> Mux/3, Mux1/2, Mux4/2
  Observer/1 -> Sum1/1, Demux/1
  Demux/6 -> Mux6/1
  theta_1/1 -> Mux1/1, Mux3/2, Mux/2
  Mux3/1 -> Scope1/1
  theta_2_dot/1 -> Mux6/2, Mux1/4, Mux/5
  Mux6/1 -> Scope1/4
  theta_2/1 -> Sum2/2, Mux1/3, Mux5/2, Mux/4
  Demux/4 -> Mux4/1
  Demux/2 -> Terminator1/1
  Demux/5 -> Mux5/1

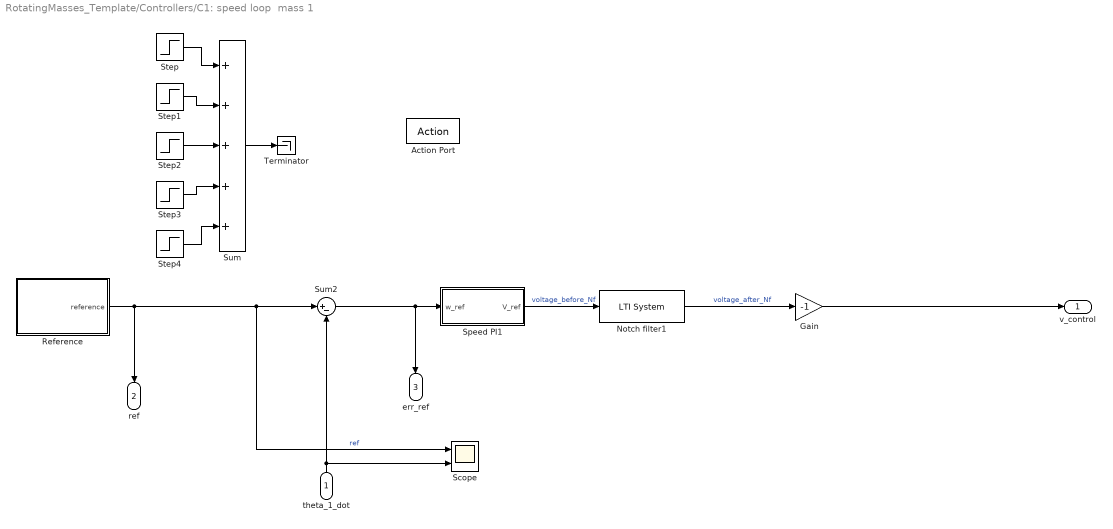
== system RotatingMasses_Template/Controllers/C1: speed loop  mass 1 ==
  theta_1_dot : Inport
  Action Port : ActionPort  ActionPortLabel=elseif(u1 == 1)
  Gain : Gain  Gain=-1
  Notch filter1 : cstblocks/LTI System  sys=controller.c1.Nf  IC=[]
  Reference : Subsystem
  Scope : Scope  NumInputPorts=2
  Speed PI1 : Subsystem
  Step : Step  After=-17  SampleTime=0
  Step1 : Step  Time=7  After=+34  SampleTime=0
  Step2 : Step  Time=13  After=-17  SampleTime=0
  Step3 : Step  Time=18  After=10  SampleTime=0
  Step4 : Step  Time=23  After=-10  SampleTime=0
  Sum : Sum  Inputs=+++++
  Sum2 : Sum  Inputs=|+-
  Terminator : Terminator
  v_control : Outport
  "ref " : Outport  Port=2
  "err_ref " : Outport  Port=3
  wires:
  theta_1_dot/1 -> Scope/2, Sum2/2
  Speed PI1/1(V_ref) -> Notch filter1/1  "voltage_before_Nf"
  Notch filter1/1 -> Gain/1  "voltage_after_Nf"
  Sum2/1 -> Speed PI1/1(w_ref), "err_ref "/1
  Gain/1 -> v_control/1
  Sum/1 -> Terminator/1
  Step/1 -> Sum/1
  Step1/1 -> Sum/2
  Step2/1 -> Sum/3
  Step3/1 -> Sum/4
  Step4/1 -> Sum/5
  Reference/1(reference) -> Scope/1, Sum2/1, "ref "/1  "ref"

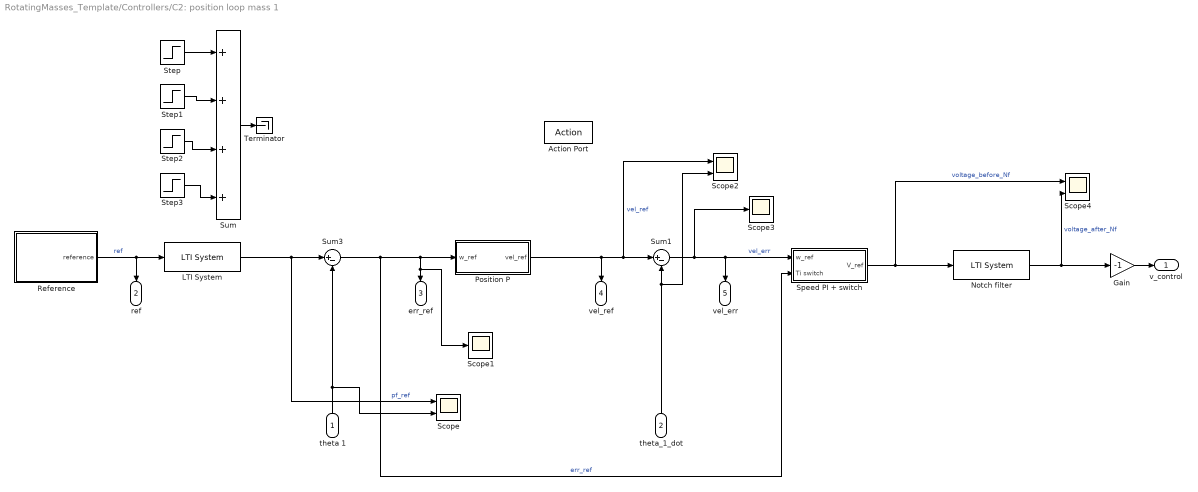
== system RotatingMasses_Template/Controllers/C2: position loop mass 1 ==
  theta 1 : Inport
  theta_1_dot : Inport  Port=2
  Action Port : ActionPort  ActionPortLabel=elseif( u1 == 2)
  Gain : Gain  Gain=-1
  LTI System : cstblocks/LTI System  sys=controller.c2.Pf  IC=[]
  Notch filter : cstblocks/LTI System  sys=controller.c2.Nf  IC=[]
  Position P : Subsystem
  Reference : Subsystem
  Scope : Scope  NumInputPorts=2
  Scope1 : Scope
  Scope2 : Scope  NumInputPorts=2
  Scope3 : Scope
  Scope4 : Scope  NumInputPorts=2
  Speed PI + switch : Subsystem
  Step : Step  After=pi/4  SampleTime=0
  Step1 : Step  Time=10  After=-2*pi-pi/4  SampleTime=0
  Step2 : Step  Time=20  After=2*pi  SampleTime=0
  Step3 : Step  Time=30  After=6*pi  SampleTime=0
  Sum : Sum  Inputs=++++
  Sum1 : Sum  Inputs=|+-
  Sum3 : Sum  Inputs=|+-
  Terminator : Terminator
  v_control : Outport
  "ref " : Outport  Port=2
  "err_ref " : Outport  Port=3
  "vel_ref " : Outport  Port=4
  "vel_err " : Outport  Port=5
  wires:
  Position P/1(vel_ref) -> Scope2/1, Sum1/1, "vel_ref "/1  "vel_ref"
  Sum1/1 -> Scope3/1, "vel_err "/1, Speed PI + switch/1(w_ref)  "vel_err"
  theta_1_dot/1 -> Scope2/2, Sum1/2
  Sum3/1 -> Scope1/1, "err_ref "/1, Position P/1(w_ref), Speed PI + switch/2("Ti switch ")  "err_ref"
  theta 1/1 -> Scope/2, Sum3/2
  Notch filter/1 -> Scope4/2, Gain/1  "voltage_after_Nf"
  Speed PI + switch/1(V_ref) -> Scope4/1, Notch filter/1  "voltage_before_Nf"
  Gain/1 -> v_control/1
  Step3/1 -> Sum/4
  Step1/1 -> Sum/2
  Step/1 -> Sum/1
  Step2/1 -> Sum/3
  Reference/1(reference) -> LTI System/1, "ref "/1  "ref"
  LTI System/1 -> Scope/1, Sum3/1  "pf_ref"
  Sum/1 -> Terminator/1

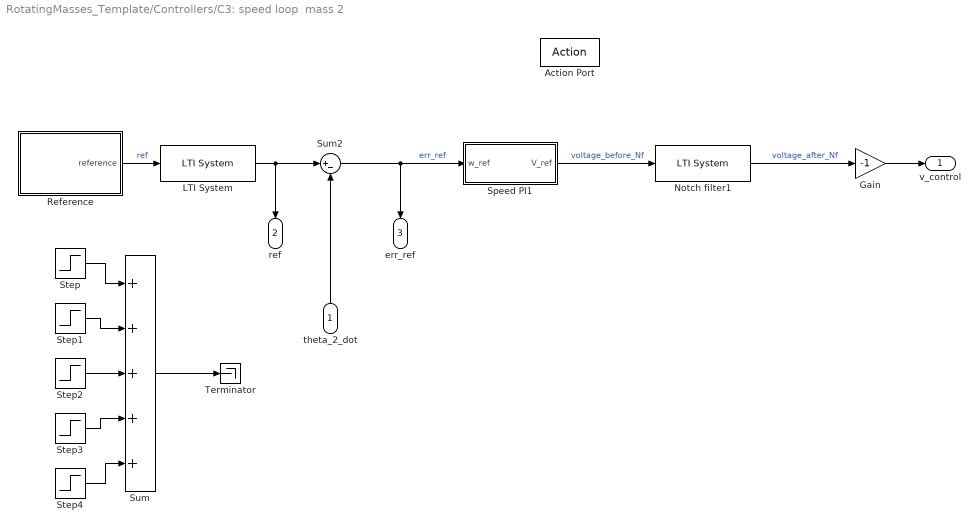
== system RotatingMasses_Template/Controllers/C3: speed loop  mass 2 ==
  theta_2_dot : Inport
  Action Port : ActionPort  ActionPortLabel=elseif( u1 == 3)
  Gain : Gain  Gain=-1
  LTI System : cstblocks/LTI System  sys=controller.c3.Pf  IC=[]
  Notch filter1 : cstblocks/LTI System  sys=controller.c3.Nf  IC=[]
  Reference : Subsystem
  Speed PI1 : Subsystem
  Step : Step  After=-17  SampleTime=0
  Step1 : Step  Time=14  After=+34  SampleTime=0
  Step2 : Step  Time=28  After=-17  SampleTime=0
  Step3 : Step  Time=42  After=10  SampleTime=0
  Step4 : Step  Time=56  After=-10  SampleTime=0
  Sum : Sum  Inputs=+++++
  Sum2 : Sum  Inputs=|+-
  Terminator : Terminator
  v_control : Outport
  "ref " : Outport  Port=2
  "err_ref " : Outport  Port=3
  wires:
  theta_2_dot/1 -> Sum2/2
  Speed PI1/1(V_ref) -> Notch filter1/1  "voltage_before_Nf"
  Notch filter1/1 -> Gain/1  "voltage_after_Nf"
  Sum2/1 -> Speed PI1/1(w_ref), "err_ref "/1  "err_ref"
  Gain/1 -> v_control/1
  Step3/1 -> Sum/4
  Step1/1 -> Sum/2
  Step/1 -> Sum/1
  Step2/1 -> Sum/3
  Step4/1 -> Sum/5
  Reference/1(reference) -> LTI System/1  "ref"
  Sum/1 -> Terminator/1
  LTI System/1 -> Sum2/1, "ref "/1

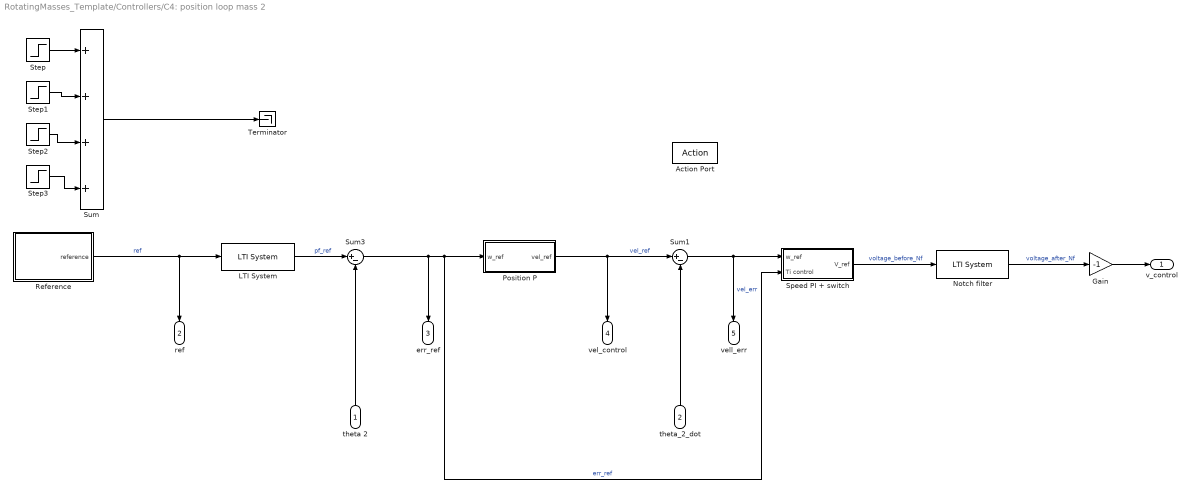
== system RotatingMasses_Template/Controllers/C4: position loop mass 2 ==
  theta 2 : Inport
  theta_2_dot : Inport  Port=2
  Action Port : ActionPort  ActionPortLabel=elseif( u1 == 4)
  Gain : Gain  Gain=-1
  LTI System : cstblocks/LTI System  sys=controller.c4.Pf  IC=[]
  Notch filter : cstblocks/LTI System  sys=controller.c4.Nf  IC=[]
  Position P : Subsystem
  Reference : Subsystem
  Speed PI + switch : Subsystem
  Step : Step  After=pi/4  SampleTime=0
  Step1 : Step  Time=10  After=-2*pi-pi/4  SampleTime=0
  Step2 : Step  Time=20  After=2*pi  SampleTime=0
  Step3 : Step  Time=30  After=6*pi  SampleTime=0
  Sum : Sum  Inputs=++++
  Sum1 : Sum  Inputs=|+-
  Sum3 : Sum  Inputs=|+-
  Terminator : Terminator
  v_control : Outport
  ref : Outport  Port=2
  err_ref : Outport  Port=3
  vel_control : Outport  Port=4
  "vell_err " : Outport  Port=5
  wires:
  Position P/1(vel_ref) -> vel_control/1, Sum1/1  "vel_ref"
  Sum1/1 -> Speed PI + switch/1(w_ref), "vell_err "/1  "vel_err"
  theta_2_dot/1 -> Sum1/2
  Sum3/1 -> Speed PI + switch/2(Ti control), Position P/1(w_ref), err_ref/1  "err_ref"
  theta 2/1 -> Sum3/2
  Notch filter/1 -> Gain/1  "voltage_after_Nf"
  Speed PI + switch/1(V_ref) -> Notch filter/1  "voltage_before_Nf"
  Step2/1 -> Sum/3
  Step1/1 -> Sum/2
  Step/1 -> Sum/1
  Step3/1 -> Sum/4
  Reference/1(reference) -> LTI System/1, ref/1  "ref"
  Gain/1 -> v_control/1
  LTI System/1 -> Sum3/1  "pf_ref"
  Sum/1 -> Terminator/1

== system RotatingMasses_Template/Controllers/C5: speed loop  mass 1 ==
  theta_1_dot : Inport
  Action Port : ActionPort  ActionPortLabel=elseif( u1 == 5)
  LTI System : cstblocks/LTI System  sys=controller.c5.Pf  IC=[]
  Notch filter1 : cstblocks/LTI System  sys=controller.c5.Nf  IC=[]
  PID Controller : simulink/Continuous/PID Controller  Controller=PID  Form=Parallel  TimeDomain=Continuous-time  SampleTime=-1  IntegratorMethod=Forward Euler  FilterMethod=Forward Euler  ControllerParametersSource=internal  P=controller.c5.Kp  I=controller.c5.Ki  D=controller.c5.Kd  UseFilter=on  N=100  TunerSelectOption=Transfer Function Based (PID Tuner App)  InitialConditionSource=internal  InitialConditionForIntegrator=0  InitialConditionForFilter=0  DifferentiatorICPrevScaledInput=0  ExternalReset=none  TrackingMode=off  Kt=1  LimitOutput=on  UpperSaturationLimit=10  LowerSaturationLimit=-10  LinearizeAsGain=on  AntiWindupMode=clamping  Kb=1  POutMin=[]  POutMax=[]  IOutMin=[]  IOutMax=[]  DOutMin=[]  DOutMax=[]  NOutMin=[]  NOutMax=[]  SumOutMin=[]  SumOutMax=[]  SaturationOutMin=[]  SaturationOutMax=[]  PParamMin=[]  PParamMax=[]  IParamMin=[]  IParamMax=[]  DParamMin=[]  DParamMax=[]  NParamMin=[]  NParamMax=[]  KbParamMin=[]  KbParamMax=[]  KtParamMin=[]  KtParamMax=[]  KbOutMin=[]  KbOutMax=[]  KtOutMin=[]  KtOutMax=[]  IntegratorOutMin=[]  IntegratorOutMax=[]  FilterOutMin=[]  FilterOutMax=[]  SumI1OutMin=[]  SumI1OutMax=[]  SumI2OutMin=[]  SumI2OutMax=[]  SumI3OutMin=[]  SumI3OutMax=[]  SumI4OutMin=[]  SumI4OutMax=[]  SumDOutMin=[]  SumDOutMax=[]  DifferentiatorOutMin=[]  DifferentiatorOutMax=[]  FilterDiffOutCoefMin=[]  FilterDiffOutCoefMax=[]  ReciprocalOutMin=[]  ReciprocalOutMax=[]  SumDenOutMin=[]  SumDenOutMax=[]  SumNumOutMin=[]  SumNumOutMax=[]  DivideOutMin=[]  DivideOutMax=[]  IntegratorContinuousStateAttributes=''  IntegratorStateMustResolveToSignalObject=off  IntegratorRTWStateStorageClass=Auto  FilterContinuousStateAttributes=''  FilterStateMustResolveToSignalObject=off  FilterRTWStateStorageClass=Auto  ParallelPVariant=InternalParameters  IdealPVariant=Disabled  IVariant=InternalParameters  DVariant=InternalParameters  IntegratorVariant=Continuous  SatVariant=Enabled  AWVariant=ContClampingParallel  PCopyVariant=Disabled  TRVariant=Disabled  FdbkBlocksVariant=Forward  IdealPFdbkVariant=Disabled  SatFdbkVariant=Disabled  DerivativeFilterVariant=ContFilter  NVariant=InternalParameters  NCopyVariant=Disabled  FilterICVariant=InternalICsFilter  IntegratorICVariant=InternalICs  ExternalResetVariant=Disabled  TRSumVariant=Passthrough  SumFdbkVariant=Disabled  SumVariant=Sum_PID
  Reference : Subsystem
  Step : Step  After=-17  SampleTime=0
  Step1 : Step  Time=14  After=+34  SampleTime=0
  Step2 : Step  Time=28  After=-17  SampleTime=0
  Step3 : Step  Time=42  After=10  SampleTime=0
  Step4 : Step  Time=56  After=-10  SampleTime=0
  Sum : Sum  Inputs=+++++
  Sum2 : Sum  Inputs=|+-
  Terminator : Terminator
  v_control : Outport
  "ref " : Outport  Port=2
  "err_ref " : Outport  Port=3
  wires:
  theta_1_dot/1 -> Sum2/2
  Notch filter1/1 -> v_control/1  "voltage_after_Nf"
  Sum2/1 -> "err_ref "/1, PID Controller/1  "err_ref"
  Step3/1 -> Sum/4
  Step1/1 -> Sum/2
  Step/1 -> Sum/1
  Step2/1 -> Sum/3
  Step4/1 -> Sum/5
  LTI System/1 -> Sum2/1  "pf_ref"
  PID Controller/1 -> Notch filter1/1  "voltage_after_PID"
  Sum/1 -> Terminator/1
  Reference/1(reference) -> "ref "/1, LTI System/1  "ref"

== system RotatingMasses_Template/Controllers/C6: speed loop  mass 2 ==
  theta_2_dot : Inport
  Action Port : ActionPort  ActionPortLabel=elseif( u1 ==6)
  LTI System : cstblocks/LTI System  sys=controller.c6.Pf  IC=[]
  Notch filter1 : cstblocks/LTI System  sys=controller.c6.Nf  IC=[]
  PID Controller : simulink/Continuous/PID Controller  Controller=PID  Form=Parallel  TimeDomain=Continuous-time  SampleTime=-1  IntegratorMethod=Forward Euler  FilterMethod=Forward Euler  ControllerParametersSource=internal  P=controller.c6.Kp  I=controller.c6.Ki  D=controller.c6.Kd  UseFilter=on  N=100  TunerSelectOption=Transfer Function Based (PID Tuner App)  InitialConditionSource=internal  InitialConditionForIntegrator=0  InitialConditionForFilter=0  DifferentiatorICPrevScaledInput=0  ExternalReset=none  TrackingMode=off  Kt=1  LimitOutput=on  UpperSaturationLimit=10  LowerSaturationLimit=-10  LinearizeAsGain=on  AntiWindupMode=clamping  Kb=1  POutMin=[]  POutMax=[]  IOutMin=[]  IOutMax=[]  DOutMin=[]  DOutMax=[]  NOutMin=[]  NOutMax=[]  SumOutMin=[]  SumOutMax=[]  SaturationOutMin=[]  SaturationOutMax=[]  PParamMin=[]  PParamMax=[]  IParamMin=[]  IParamMax=[]  DParamMin=[]  DParamMax=[]  NParamMin=[]  NParamMax=[]  KbParamMin=[]  KbParamMax=[]  KtParamMin=[]  KtParamMax=[]  KbOutMin=[]  KbOutMax=[]  KtOutMin=[]  KtOutMax=[]  IntegratorOutMin=[]  IntegratorOutMax=[]  FilterOutMin=[]  FilterOutMax=[]  SumI1OutMin=[]  SumI1OutMax=[]  SumI2OutMin=[]  SumI2OutMax=[]  SumI3OutMin=[]  SumI3OutMax=[]  SumI4OutMin=[]  SumI4OutMax=[]  SumDOutMin=[]  SumDOutMax=[]  DifferentiatorOutMin=[]  DifferentiatorOutMax=[]  FilterDiffOutCoefMin=[]  FilterDiffOutCoefMax=[]  ReciprocalOutMin=[]  ReciprocalOutMax=[]  SumDenOutMin=[]  SumDenOutMax=[]  SumNumOutMin=[]  SumNumOutMax=[]  DivideOutMin=[]  DivideOutMax=[]  IntegratorContinuousStateAttributes=''  IntegratorStateMustResolveToSignalObject=off  IntegratorRTWStateStorageClass=Auto  FilterContinuousStateAttributes=''  FilterStateMustResolveToSignalObject=off  FilterRTWStateStorageClass=Auto  ParallelPVariant=InternalParameters  IdealPVariant=Disabled  IVariant=InternalParameters  DVariant=InternalParameters  IntegratorVariant=Continuous  SatVariant=Enabled  AWVariant=ContClampingParallel  PCopyVariant=Disabled  TRVariant=Disabled  FdbkBlocksVariant=Forward  IdealPFdbkVariant=Disabled  SatFdbkVariant=Disabled  DerivativeFilterVariant=ContFilter  NVariant=InternalParameters  NCopyVariant=Disabled  FilterICVariant=InternalICsFilter  IntegratorICVariant=InternalICs  ExternalResetVariant=Disabled  TRSumVariant=Passthrough  SumFdbkVariant=Disabled  SumVariant=Sum_PID
  Reference : Subsystem
  Step : Step  After=-17  SampleTime=0
  Step1 : Step  Time=14  After=+34  SampleTime=0
  Step2 : Step  Time=28  After=-17  SampleTime=0
  Step3 : Step  Time=42  After=10  SampleTime=0
  Step4 : Step  Time=56  After=-10  SampleTime=0
  Sum : Sum  Inputs=+++++
  Sum2 : Sum  Inputs=|+-
  Terminator : Terminator
  v_control : Outport
  "ref " : Outport  Port=2
  "err_ref " : Outport  Port=3
  wires:
  theta_2_dot/1 -> Sum2/2
  PID Controller/1 -> Notch filter1/1  "voltage_after_PID"
  Notch filter1/1 -> v_control/1  "voltage_after_Nf"
  Sum2/1 -> "err_ref "/1, PID Controller/1  "err_ref"
  Step3/1 -> Sum/4
  Step1/1 -> Sum/2
  Step/1 -> Sum/1
  Step2/1 -> Sum/3
  Step4/1 -> Sum/5
  LTI System/1 -> Sum2/1  "pf_ref"
  Sum/1 -> Terminator/1
  Reference/1(reference) -> LTI System/1, "ref "/1  "ref"
